simulink model "TANK1"  (Simulink 3.00)
settings: Solver=ode45  SolverMode=SingleTasking  StartTime=0.0  StopTime=200  MaxStep=.10  RelTol=1e-4  AbsTol=1e-4
CloseFcn:
  | ;slview('closediagram',bdroot);;slview('closediagram',bdroot);
settings Model: TimeSaveName=t  SaveOutput=off

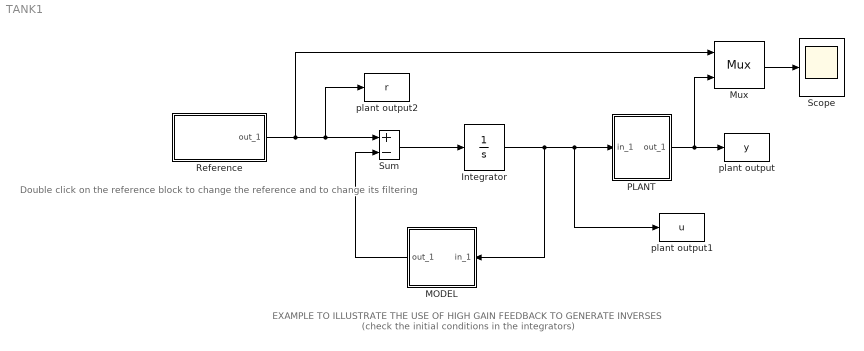
== system TANK1 ==
  note: EXAMPLE TO ILLUSTRATE THE USE OF HIGH GAIN FEEDBACK TO GENERATE INVERSES
      | (check  the initial conditions in the integrators)
  note: Double click on the reference
      |  block to change the
      | reference and to change its filtering
  Integrator : Integrator  ExternalReset=none  InitialConditionSource=internal  InitialCondition=2  LimitOutput=off  UpperSaturationLimit=inf  LowerSaturationLimit=-inf  ShowSaturationPort=off  ShowStatePort=off  AbsoluteTolerance=auto
  MODEL : Subsystem  Orientation=left
      mask Type: Model
      mask Display: disp('Model')
  Mux : Mux  Inputs=2
      settings: DisplayOption=none
  PLANT : Subsystem
      mask Display: disp('Plant')
  "Reference " : Subsystem
      mask Type: Ref
      mask Display: disp('Reference')
  Scope : Scope
      settings: TickLabels=on  TimeRange=200.000000  YMin=-2  YMax=2  SaveToWorkspace=off  SaveName=ScopeData  DataFormat=Matrix
  Sum : Sum  Inputs=+-  SaturateOnIntegerOverflow=on
  plant output : ToWorkspace  VariableName=y  SampleTime=0  SaveFormat=Matrix
      settings: Buffer=6000
  plant output1 : ToWorkspace  VariableName=u  SampleTime=0  SaveFormat=Matrix
      settings: Buffer=6000
  plant output2 : ToWorkspace  VariableName=r  SampleTime=0  SaveFormat=Matrix
      settings: Buffer=6000
  wires:
  Sum/1 -> Integrator/1
  Mux/1 -> Scope/1
  MODEL/1(out_1) -> Sum/2
  "Reference "/1(out_1) -> Mux/1, Sum/1, plant output2/1
  Integrator/1 -> MODEL/1(in_1), PLANT/1(in_1), plant output1/1
  PLANT/1(out_1) -> plant output/1, Mux/2

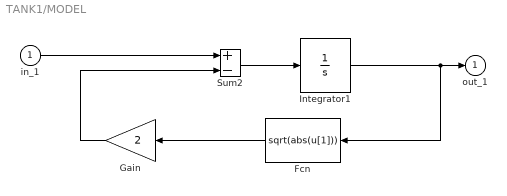
== system TANK1/MODEL ==
  in_1 : Inport  Port=1  PortWidth=-1  SampleTime=-1  DataType=auto
      settings: SignalType=auto
  Fcn : Fcn  Orientation=left  Expr=sqrt(abs(u[1]))
  Gain : Gain  Orientation=left  Gain=2  SaturateOnIntegerOverflow=on
  Integrator1 : Integrator  ExternalReset=none  InitialConditionSource=internal  InitialCondition=0.25  LimitOutput=off  UpperSaturationLimit=inf  LowerSaturationLimit=-inf  ShowSaturationPort=off  ShowStatePort=off  AbsoluteTolerance=auto
  Sum2 : Sum  Inputs=+-  SaturateOnIntegerOverflow=on
  out_1 : Outport  Port=1  InitialOutput=0
  wires:
  Sum2/1 -> Integrator1/1
  Fcn/1 -> Gain/1
  Gain/1 -> Sum2/2
  in_1/1 -> Sum2/1
  Integrator1/1 -> out_1/1, Fcn/1

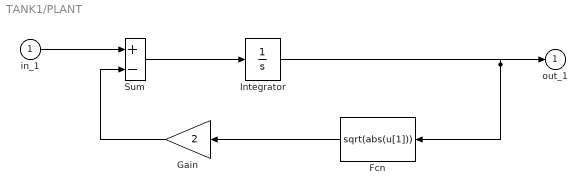
== system TANK1/PLANT ==
  in_1 : Inport  Port=1  PortWidth=-1  SampleTime=-1  DataType=auto
      settings: SignalType=auto
  Fcn : Fcn  Orientation=left  Expr=sqrt(abs(u[1]))
  Gain : Gain  Orientation=left  Gain=2  SaturateOnIntegerOverflow=on
  Integrator : Integrator  ExternalReset=none  InitialConditionSource=internal  InitialCondition=0.25  LimitOutput=off  UpperSaturationLimit=inf  LowerSaturationLimit=-inf  ShowSaturationPort=off  ShowStatePort=off  AbsoluteTolerance=auto
  Sum : Sum  Inputs=+-  SaturateOnIntegerOverflow=on
  out_1 : Outport  Port=1  InitialOutput=0
  wires:
  Sum/1 -> Integrator/1
  Gain/1 -> Sum/2
  in_1/1 -> Sum/1
  Integrator/1 -> out_1/1, Fcn/1
  Fcn/1 -> Gain/1

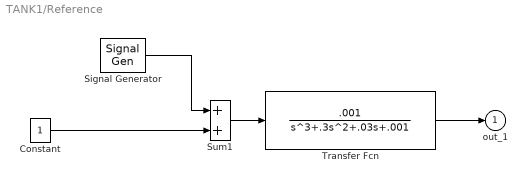
== system TANK1/Reference  ==
  Constant : Constant  Value=1
  Signal Generator : SignalGenerator  WaveForm=square  Amplitude=0.500000  Frequency=0.100000  Units=rad/sec
  Sum1 : Sum  Inputs=++  SaturateOnIntegerOverflow=on
  Transfer Fcn : TransferFcn  Numerator=[.001]  Denominator=[1 .3 .03 .001]
  out_1 : Outport  Port=1  InitialOutput=0
  wires:
  Sum1/1 -> Transfer Fcn/1
  Signal Generator/1 -> Sum1/1
  Constant/1 -> Sum1/2
  Transfer Fcn/1 -> out_1/1
